simulink model "EarlyReturn9_2018a"  (R2018a)
settings: Solver=VariableStepAuto  StartTime=0.0  StopTime=0.1  RelTol=1e-3
settings Model: Creator=BEAR  LastModifiedBy=apple

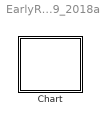
== system EarlyReturn9_2018a ==
  Chart : Stateflow chart  TreatAsAtomicUnit=on

== stateflow chart EarlyReturn9_2018a/Chart ==
  state A
    en: fprintf("en_A")
    ex: fprintf("ex_A")
    state A1
      en: fprintf("en_A1")
      ex: fprintf("ex_A1")
    state A2
      en: fprintf("en_A2")
      ex: fprintf("ex_A2")
    (default) -> A1
    A1 -> (junction 12) : {fprintf("pre")}
    (junction 12) -> A2 : {E;fprintf("E")}
  state B
    en: fprintf("en_B")
    ex: fprintf("ex_B")
  (default) -> A
  A -> B : E
  events: E local FUNCTION_CALL_EVENT
